simulink model "Simulation"  (R2023a)
settings: Solver=ode4  StartTime=0.0  StopTime=25  FixedStep=0.0001  RelTol=1e-6
settings Model: Creator=Ahmed  LastModifiedBy=Ahmed

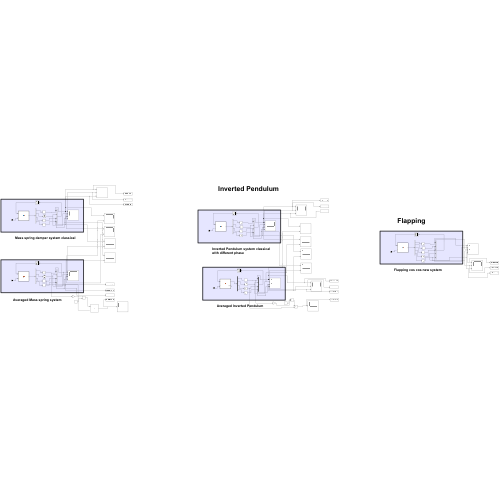
[thumbnail: Simulink's stored preview of the top-level diagram]
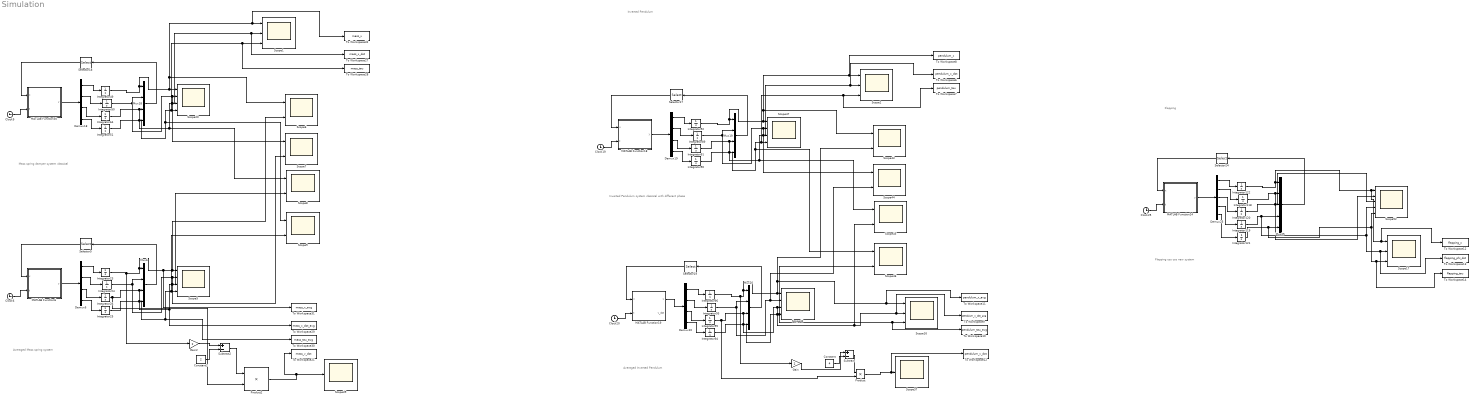
== system Simulation ==
  note: Inverted Pendulum
  note: Mass spring damper system classical
  note: Averaged Mass spring system
  note: Inverted Pendulum system classical with different phase
  note: Averaged Inverted Pendulum
  note: Flapping cos cos new system
  note: Flapping
  Clock{6,9,19..20,25} (5 alike) : Clock
  Constant : Constant  Value=4
  Constant2 : Constant  Value=2
  Demux{6,18..20} (4 alike) : Demux
  Demux25 : Demux  Outputs=5
  Gain : Gain  Gain=2
  Gain2 : Gain  Gain=2
  Integrator{24..26,50..51,64,89..96,118..122} (19 alike) : Integrator
  Integrator23 : Integrator  InitialCondition=3
  Integrator49 : Integrator  InitialCondition=3
  MATLAB Function18 : MATLAB Function  TreatAsAtomicUnit=on
  MATLAB Function19 : MATLAB Function  TreatAsAtomicUnit=on
  MATLAB Function24 : MATLAB Function  TreatAsAtomicUnit=on
  MATLAB Function30 : MATLAB Function  TreatAsAtomicUnit=on
  MATLAB Function6 : MATLAB Function  TreatAsAtomicUnit=on
  Mux{6,18..20} (4 alike) : Mux
  Mux25 : Mux  Inputs=5
  Product : Product
  Product2 : Product
  Scope{1..2,16..17} (4 alike) : Scope  NumInputPorts=3
  Scope{5,20,42,47} (4 alike) : Scope  NumInputPorts=4
  Scope37 : Scope
  Scope39 : Scope
  Scope{6..9,43..46} (8 alike) : Scope  NumInputPorts=2
  Scope52 : Scope  NumInputPorts=5
  Selector{5,17..19} (4 alike) : Selector  InputPortWidth=4  IndexOptions=Index vector (dialog)  Indices=[1 2 3 4]  OutputSizes=1
  Selector24 : Selector  InputPortWidth=5  IndexOptions=Index vector (dialog)  Indices=[1 2 3 4 5]  OutputSizes=1
  Subtract : Sum  Inputs=+-
  Subtract2 : Sum  Inputs=+-
  To Workspace10 : ToWorkspace  VariableName=pendulum_tau_avg  SaveFormat=Timeseries  SampleTime=-1
  To Workspace11 : ToWorkspace  VariableName=pendulum_x_avg  SaveFormat=Timeseries  SampleTime=-1
  To Workspace12 : ToWorkspace  VariableName=flapping_z  SampleTime=-1
      settings: Save2DSignal=2-D array (concatenate along first dimension)
  To Workspace13 : ToWorkspace  VariableName=flapping_phi_dot  SampleTime=-1
      settings: Save2DSignal=2-D array (concatenate along first dimension)
  To Workspace14 : ToWorkspace  VariableName=flapping_tau  SampleTime=-1
      settings: Save2DSignal=2-D array (concatenate along first dimension)
  To Workspace21 : ToWorkspace  VariableName=mass_v_dot  SaveFormat=Timeseries  SampleTime=-1
  To Workspace22 : ToWorkspace  VariableName=pendulum_v_dot  SaveFormat=Timeseries  SampleTime=-1
  To Workspace27 : ToWorkspace  VariableName=mass_x_dot  SaveFormat=Timeseries  SampleTime=-1
  To Workspace28 : ToWorkspace  VariableName=mass_tau  SaveFormat=Timeseries  SampleTime=-1
  To Workspace29 : ToWorkspace  VariableName=mass_x_dot_avg  SaveFormat=Timeseries  SampleTime=-1
  To Workspace30 : ToWorkspace  VariableName=mass_tau_avg  SaveFormat=Timeseries  SampleTime=-1
  To Workspace31 : ToWorkspace  VariableName=mass_x_avg  SaveFormat=Timeseries  SampleTime=-1
  To Workspace32 : ToWorkspace  VariableName=mass_x  SaveFormat=Timeseries  SampleTime=-1
  To Workspace6 : ToWorkspace  VariableName=pendulum_x_dot  SaveFormat=Timeseries  SampleTime=-1
  To Workspace7 : ToWorkspace  VariableName=pendulum_tau  SaveFormat=Timeseries  SampleTime=-1
  To Workspace8 : ToWorkspace  VariableName=pendulum_x  SaveFormat=Timeseries  SampleTime=-1
  To Workspace9 : ToWorkspace  VariableName=pendulum_x_dot_avg  SaveFormat=Timeseries  SampleTime=-1
  wires:
  Integrator25/1 -> Mux6/4, To Workspace30/1, Scope5/4, Scope9/2
  Clock6/1 -> MATLAB Function6/2(t)
  Demux18/1 -> Integrator49/1
  MATLAB Function30/1(y) -> Demux18/1
  Demux18/3 -> Integrator64/1
  Demux6/3 -> Integrator26/1
  Integrator23/1 -> Gain2/1, To Workspace31/1, Scope6/2, Scope5/1, Mux6/1
  Demux6/1 -> Integrator23/1
  Demux6/4 -> Integrator25/1
  Mux6/1 -> Selector5/1
  Selector5/1 -> MATLAB Function6/1(x)
  Integrator24/1 -> Mux6/2, Scope7/2, Scope5/2
  Demux18/2 -> Integrator50/1
  Demux6/2 -> Integrator24/1
  Integrator51/1 -> Scope20/4, To Workspace28/1, Scope1/3, Scope9/1, Mux18/4
  Clock9/1 -> MATLAB Function30/2(t)
  Mux18/1 -> Selector18/1
  Integrator64/1 -> Scope8/1, To Workspace27/1, Scope1/2, Scope20/3, Mux18/3
  MATLAB Function6/1(y) -> Demux6/1
  Selector18/1 -> MATLAB Function30/1(x)
  Integrator49/1 -> Mux18/1, Scope6/1, To Workspace32/1, Scope1/1, Scope20/1
  Demux18/4 -> Integrator51/1
  Integrator26/1 -> Product2/2, Mux6/3, Scope8/2, Scope5/3, To Workspace29/1
  Integrator50/1 -> Scope7/1, Scope20/2, Mux18/2
  Integrator94/1 -> Mux20/4, Scope46/2, To Workspace10/1, Scope16/3, Scope42/4
  Clock20/1 -> MATLAB Function19/2(t)
  Demux19/1 -> Integrator92/1
  Mux20/1 -> Selector19/1
  Integrator89/1 -> Scope47/2, Scope44/1, Mux19/2
  Demux19/4 -> Integrator90/1
  Demux20/4 -> Integrator94/1
  Mux19/1 -> Selector17/1
  Integrator91/1 -> Scope45/1, To Workspace6/1, Scope2/2, Scope47/3, Mux19/3
  Integrator90/1 -> Scope47/4, To Workspace7/1, Scope2/3, Scope46/1, Mux19/4
  Demux19/2 -> Integrator89/1
  Integrator92/1 -> Mux19/1, Scope43/1, To Workspace8/1, Scope2/1, Scope47/1
  Demux20/3 -> Integrator95/1
  Integrator96/1 -> Scope43/2, To Workspace11/1, Scope16/1, Scope42/1, Mux20/1, Gain/1
  Demux19/3 -> Integrator91/1
  Integrator93/1 -> Mux20/2, Scope42/2, Scope44/2
  Integrator95/1 -> Product/2, Mux20/3, Scope45/2, To Workspace9/1, Scope16/2, Scope42/3
  Demux20/2 -> Integrator93/1
  MATLAB Function18/1(y) -> Demux19/1
  Selector19/1 -> MATLAB Function19/1(x)
  Demux20/1 -> Integrator96/1
  Clock19/1 -> MATLAB Function18/2(t)
  Selector17/1 -> MATLAB Function18/1(x)
  MATLAB Function19/1(y) -> Demux20/1
  Clock25/1 -> MATLAB Function24/2(t)
  Integrator118/1 -> Mux25/2, Scope52/2
  Integrator119/1 -> Mux25/4, To Workspace13/1, Scope17/2, Scope52/4
  Selector24/1 -> MATLAB Function24/1(x)
  Integrator122/1 -> Mux25/1, To Workspace12/1, Scope17/1, Scope52/1
  Demux25/1 -> Integrator122/1
  Integrator120/1 -> Mux25/3, Scope52/3
  MATLAB Function24/1(y) -> Demux25/1
  Demux25/4 -> Integrator119/1
  Demux25/3 -> Integrator120/1
  Demux25/2 -> Integrator118/1
  Demux25/5 -> Integrator121/1
  Mux25/1 -> Selector24/1
  Integrator121/1 -> Mux25/5, To Workspace14/1, Scope17/3, Scope52/5
  Gain/1 -> Subtract/1
  Constant/1 -> Subtract/2
  Subtract/1 -> Product/1
  Product/1 -> To Workspace22/1, Scope37/1
  Gain2/1 -> Subtract2/1
  Constant2/1 -> Subtract2/2
  Product2/1 -> To Workspace21/1, Scope39/1
  Subtract2/1 -> Product2/1

== matlab function Simulation/MATLAB Function6 ==
  data: x input; y output; t input
function y = fcn(x,t)
% Parameters for mass-spring-damper system
m = 1; % Mass
k = 20; % Spring constant
c = 2; % Damping coefficient
% Define the system of equations as a function
omega=50;
kk=5;
J=(x(1)-3)^2;
phi_0=0;


c1=3;
a1=0.3;

y = [
    x(3); % dx1/dt = x2 (velocity)
    x(4)
    -(k/m) * x(1) - (c/m) * x(3) + (1/m) * x(4)* c1; % dx2/dt = acceleration with damping, spring force, and control input
    -(0.5*kk*a1)*(2*x(1)-2)
];

== matlab function Simulation/MATLAB Function18 ==
  data: x input; y output; t input
function y = fcn(x,t)

% Parameters for mass-spring-damper system
m = 1; % Mass of the pendulum bob (kg)
L = 1; % Length of the pendulum rod (m)
g = 9.81; % Gravitational acceleration (m/s^2)
beta = 10; % Damping coefficient (Ns/m)
% Define the system of equations as a function

c1=1;
a1=0.5;
omega=50;
k=2;
J=(x(1)-2)^2;


y = [
    x(3); % dx1/dt = x2 (velocity)
    x(4);
    (g/L) * sin(x(1)) - (beta/(m*L)) * x(3) + c1 * x(4)+ a1*omega*cos(omega*t); % dx2/dt = acceleration with damping, spring force, and control input
    k*J*omega*cos(omega*t)
];

== matlab function Simulation/MATLAB Function19 ==
  data: x input; y output; t input; v_dot output
function [y,v_dot] = fcn(x,t)

% Parameters for mass-spring-damper system
m = 1; % Mass of the pendulum bob (kg)
L = 1; % Length of the pendulum rod (m)
g = 9.81; % Gravitational acceleration (m/s^2)
beta = 10; % Damping coefficient (Ns/m)

c1=1;
a1=0.5;
% Define the system of equations as a function


k=2;
J=(x(1)-2)^2;



y = [
    x(3); % dx1/dt = x2 (velocity)
    x(4);
    (g/L) * sin(x(1)) - (beta/(m*L)) * x(3) + c1 * x(4); % dx2/dt = acceleration with damping, spring force, and control input
    -0.5*k*(2*x(1)-4)*a1
];

%v_dot=(2*x(1)-4)*((g/L) * sin(x(1)) - (beta/(m*L)) * x(3) + c1 * x(4));


nabla_q_J = (2*x(1)-4);

% Define q_dot as a vector
q_dot = [(g/L) * sin(x(1)) - (beta/(m*L)) * x(3) + c1 * x(4) ];

% Compute v_dot using dot product
v_dot = dot(nabla_q_J, q_dot);

== matlab function Simulation/MATLAB Function24 ==
  data: x input; y output; t input
function y= fcn(x,t)

kd1 =0.0353739; %system parameter kd1
g =9.81; %system parameter g
kL =0.000621676; %system parameter kL
%a4 =1.37801*10^( -7); %system parameter I
f = 26.3; %system frequency in Hz
%T = 1/f; %system period
%a5 =2*pi*f; %system parameter omega
kd2 =0.33915; %system parameter kd2
kd3 =16.5766; %system parameter kd3

IF=1.37801*10^( -7);

omega=2*pi*f;

J=(x(1)-1)^2;


a=2.575e-05;


c1=0.15;
c2=1;
a1=a*c1;
a2=(1/IF)*a;
k=-60*(1/IF)*a;

epsilon = 50;
abs_phi_dot=x(4) * (2/pi)*atan(epsilon*x(4));

y= [x(3); 
    x(4);
    -kd1*abs(x(4))*x(3)+g-kL*x(4)^2+   c1*x(5) + a1*omega*cos(omega*t) ;
    -kd3*x(3)*x(4)-kd2*abs(x(4))*x(4)+ c2*x(5) + a2*omega*cos(omega*t);
     k*J*omega*cos(omega*t)
    ];
% AA=c2*x(5) + a2*omega*cos(omega*t);

== matlab function Simulation/MATLAB Function30 ==
  data: x input; y output; t input
function y = fcn(x,t)

% Parameters for mass-spring-damper system
m = 1; % Mass
k = 20; % Spring constant
c = 2; % Damping coefficient
% Define the system of equations as a function
omega=50;
kk=5;
J=(x(1)-1)^2;
phi_0=0;

c1=3;
a1=0.3;

y = [
    x(3); 
    x(4)
    -(k/m) * x(1) - (c/m) * x(3) + (1/m) * x(4)*c1+ a1* omega*cos(omega*t+phi_0); 
    kk*J*omega*cos(omega*t)
];
